simulink model "Control_Schematic_11"  (Simulink 8.3)
settings: Solver=ode4  StartTime=0.0  StopTime=50  FixedStep=Ts  RelTol=1e-3
values from neighbouring files (symbols this model uses):
  b = 156    [StartUp_1.m]    (also in StartUp_11_Validation.m; StartUp_3.m; StartUp_4.m; StartUp_7.m)
  r = 820    [StartUp_1.m]    (also in StartUp_11_Validation.m = 50; StartUp_3.m = 520; StartUp_4.m = 0.01; StartUp_7.m = 0.01)
  Ts = 1/1000    (= 0.001)    [StartUp_1.m]    (also in StartUp_11_Validation.m = 0.01; StartUp_3.m; StartUp_4.m; StartUp_7.m)
undefined symbols (not defined in the file or in its folder): Aob, Beta_Correction, Bob, Cob, Dob
undefined symbols (not defined in the file): ADAMS_cwd, ADAMS_exec, ADAMS_host, ADAMS_init, ADAMS_inputs, ADAMS_outputs, ADAMS_prefix, ADAMS_static, ADAMS_sysdir
libraries: cstblocks x2, simulink x1
settings Model: Creator=baqumau  LastModifiedBy=baqumau
settings DataIOCC: SignalLoggingSaveFormat=Dataset
settings DebuggingCC: UnderspecifiedInitializationDetection=Simplified  StateNameClashWarn=none
settings GRTTargetCC: CombineOutputUpdateFcns=on  GRTInterface=off

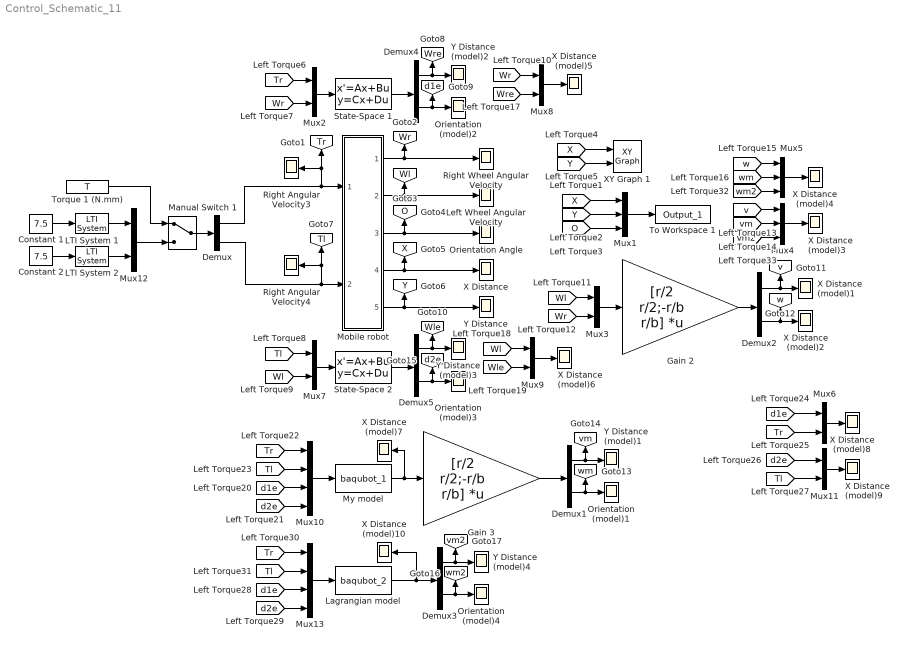
== system Control_Schematic_11 ==
  Constant 1 : Constant  Value=7.5
  Constant 2 : Constant  Value=7.5
  Demux{,1..5} (6 alike) : Demux  Outputs=2
  Gain 2 : Gain  Gain=[r/2 r/2;-r/b r/b]  Multiplication=Matrix(K*u)
  Gain 3 : Gain  Gain=[r/2 r/2;-r/b r/b]  Multiplication=Matrix(K*u)
  LTI System 1 : cstblocks/LTI System  sys=Fz  IC=[]
  LTI System 2 : cstblocks/LTI System  sys=Fz  IC=[]
  Lagrangian model : S-Function  FunctionName=baqubot_2  Parameters=par  EnableBusSupport=off
  Left Wheel Angular Velocity : Scope
      settings: YMin=-1  YMax=1  SaveName=ScopeData2
  Manual Switch 1 : ManualSwitch
  Mobile robot : Subsystem
  Mux1 : Mux  Inputs=3
  Mux10 : Mux
  Mux{2..3,6..9,11..12} (8 alike) : Mux  Inputs=2
  Mux13 : Mux
  Mux4 : Mux  Inputs=3
  Mux5 : Mux  Inputs=3
  My model : S-Function  FunctionName=baqubot_1  Parameters=par  EnableBusSupport=off
  Orientation (model){1..4} (4 alike) : Scope
      Orientation (model)1 settings: YMin=1.49226  YMax=1.64934  SaveName=ScopeData12
      Orientation (model)2 settings: YMin=-15  YMax=15  SaveName=ScopeData6
      Orientation (model)3 settings: YMin=-15  YMax=15  SaveName=ScopeData9
      Orientation (model)4 settings: YMin=1.49226  YMax=1.64934  SaveName=ScopeData23
  Orientation Angle : Scope
      settings: YMin=-4  YMax=4
  Right Angular Velocity3 : Scope
      settings: YMin=-1.5  YMax=5.5  SaveName=ScopeData7
  Right Angular Velocity4 : Scope
      settings: YMin=-25  YMax=25  SaveName=ScopeData8
  Right Wheel Angular Velocity : Scope
      settings: YMin=-1  YMax=1  SaveName=ScopeData3
  State-Space 1 : StateSpace  A=Aob  B=Bob  C=Cob  D=Dob  X0=0
  State-Space 2 : StateSpace  A=Aob  B=Bob  C=Cob  D=Dob  X0=0
  To Workspace 1 : ToWorkspace  VariableName=Output_1  SaveFormat=Structure With Time  SampleTime=-1
  Torque 1 (N.mm) : FromWorkspace  VariableName=T  SampleTime=Ts  Interpolate=off  OutputAfterFinalValue=Holding final value
  X Distance : Scope
      settings: YMin=0  YMax=5000  SaveName=ScopeData4
  X Distance (model){1..10} (10 alike) : Scope
      X Distance (model)1 settings: YMin=0  YMax=5000  SaveName=ScopeData10
      X Distance (model)10 settings: YMin=0  YMax=5000  SaveName=ScopeData22
      X Distance (model)2 settings: YMin=0  YMax=5000  SaveName=ScopeData11
      X Distance (model)3 settings: YMin=0  YMax=800  SaveName=ScopeData14
      X Distance (model)4 settings: YMin=0  YMax=5000  SaveName=ScopeData15
      X Distance (model)5 settings: YMin=0  YMax=5000  SaveName=ScopeData17
      X Distance (model)6 settings: YMin=0  YMax=5000  SaveName=ScopeData18
      X Distance (model)7 settings: YMin=0  YMax=5000  SaveName=ScopeData19
      X Distance (model)8 settings: TimeRange=35  YMin=-20  YMax=20  SaveName=ScopeData20
      X Distance (model)9 settings: YMin=-15  YMax=15  SaveName=ScopeData21
  XY Graph 1 : simulink/Sinks/XY Graph  xmin=0  xmax=5000  ymin=0  ymax=5000  st=-1
  Y Distance : Scope
      settings: YMin=0  YMax=5000
  Y Distance (model){1..4} (4 alike) : Scope
      Y Distance (model)1 settings: YMin=0  YMax=5000  SaveName=ScopeData13
      Y Distance (model)2 settings: YMin=0  YMax=5000  SaveName=ScopeData5
      Y Distance (model)3 settings: YMin=0  YMax=5000  SaveName=ScopeData16
      Y Distance (model)4 settings: YMin=0  YMax=5000  SaveName=ScopeData24
  tag scope: O=global, Tl=global, Tr=global, Wl=global, Wle=global, Wr=global, Wre=global, X=global, Y=global, d1e=global, d2e=global, v=global, vm2=global, vm=global, w=global, wm2=global, wm=global
  wires:
  Mobile robot/1(Wrw) -> Right Wheel Angular Velocity/1, [Wr]
  Mobile robot/2(Wlw) -> Left Wheel Angular Velocity/1, [Wl]
  Mobile robot/3(Alpha) -> Orientation Angle/1, [O]
  Mobile robot/4(X_Dist) -> X Distance/1, [X]
  Mobile robot/5(Y_Dist) -> Y Distance/1, [Y]
  [X] -> Mux1/1
  [Y] -> Mux1/2
  [O] -> Mux1/3
  Mux1/1 -> To Workspace 1/1
  Demux/1 -> Mobile robot/1(Trw), [Tr], Right Angular Velocity3/1
  Demux/2 -> Mobile robot/2(Tlw), [Tl], Right Angular Velocity4/1
  [X] -> XY Graph 1/1
  [Y] -> XY Graph 1/2
  [Wl] -> Mux3/1
  [Wr] -> Mux3/2
  Mux3/1 -> Gain 2/1
  Gain 2/1 -> Demux2/1
  Demux2/2 -> [w], X Distance (model)2/1
  Demux2/1 -> [v], X Distance (model)1/1
  Demux1/1 -> Y Distance (model)1/1, [vm]
  Demux1/2 -> Orientation (model)1/1, [wm]
  [vm] -> Mux4/2
  Mux4/1 -> X Distance (model)3/1
  [wm] -> Mux5/2
  Mux5/1 -> X Distance (model)4/1
  [Tr] -> Mux10/1
  Gain 3/1 -> Demux1/1
  Mux10/1 -> My model/1
  My model/1 -> X Distance (model)7/1, Gain 3/1
  Mux2/1 -> State-Space 1/1
  [Tr] -> Mux2/1
  [Wr] -> Mux2/2
  State-Space 1/1 -> Demux4/1
  Demux4/2 -> [d1e], Orientation (model)2/1
  Demux4/1 -> [Wre], Y Distance (model)2/1
  Mux7/1 -> State-Space 2/1
  [Tl] -> Mux7/1
  [Wl] -> Mux7/2
  State-Space 2/1 -> Demux5/1
  Demux5/2 -> Orientation (model)3/1, [d2e]
  Demux5/1 -> Y Distance (model)3/1, [Wle]
  [Wr] -> Mux8/1
  Mux8/1 -> X Distance (model)5/1
  [Wre] -> Mux8/2
  Mux9/1 -> X Distance (model)6/1
  [Wle] -> Mux9/2
  [Wl] -> Mux9/1
  [Tl] -> Mux10/2
  [d1e] -> Mux10/3
  [d2e] -> Mux10/4
  [d1e] -> Mux6/1
  [Tr] -> Mux6/2
  Mux6/1 -> X Distance (model)8/1
  [d2e] -> Mux11/1
  [Tl] -> Mux11/2
  Mux11/1 -> X Distance (model)9/1
  Manual Switch 1/1 -> Demux/1
  Torque 1 (N.mm)/1 -> Manual Switch 1/1
  Constant 1/1 -> LTI System 1/1
  Constant 2/1 -> LTI System 2/1
  LTI System 2/1 -> Mux12/2
  LTI System 1/1 -> Mux12/1
  Mux12/1 -> Manual Switch 1/2
  [Tr] -> Mux13/1
  Mux13/1 -> Lagrangian model/1
  [Tl] -> Mux13/2
  [d1e] -> Mux13/3
  [d2e] -> Mux13/4
  Demux3/1 -> [vm2], Y Distance (model)4/1
  Demux3/2 -> [wm2], Orientation (model)4/1
  Lagrangian model/1 -> X Distance (model)10/1, Demux3/1
  [wm2] -> Mux5/3
  [vm2] -> Mux4/3
  [w] -> Mux5/1
  [v] -> Mux4/1

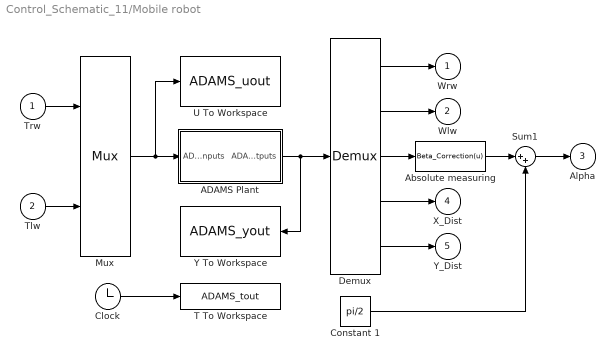
== system Control_Schematic_11/Mobile robot ==
  Trw : Inport
  Tlw : Inport  Port=2
  ADAMS Plant : Subsystem  LoadFcn=|  InitFcn=clear mex  mask(Adams Plant){exevie=ADAMS_sysdir, nam_in=ADAMS_inputs, namout=ADAMS_outputs, nampre=ADAMS_prefix, outfil=ADAMS_prefix, exesol=ADAMS_exec, stat=ADAMS_static, inicmd=[ADAMS_init], exetyp=C++, comtyp=PIPE(DDE), workdir=ADAMS_cwd, ada_host=ADAMS_host, modani=batch, modsim=discrete, dft=no, simulink_lead_cosim=yes, pin_interp_order=0, pout_extrap_order=0, pin_extrap_order=0, pout_interp_order=0, dt_out=Ts, o_rate=1, more=off}
      | %check based on dialog box setting for when setting by popup menu                                             
      | if exist('ADAMS_solver_type')                                                                                 
      |   if strcmp(ADAMS_solver_type,'C++')                                                                          
      |     set_param(gcb,'exetyp','C++');                                                                            
      |   else                                                                                                        
      |     set_param(gcb,'exetyp','Fortran');                                                                        
      |   end                                                                                                         
      | else                                                                                                          
      |   set_param(gcb,'exetyp','C++');                                                                              
      | end                                                                                                           
      | %set the mode if using acar_solver                                                                            
      | %REQUIRED HERE BECAUSE BELOW CAUSES MDLTERMINATE TO BE CALLED 2 TIMES IN MIDDLE OF SIMULATION WHEN SET IN MASK
      |                                                                                                               
      | %enable the direct feedthrough, sim mode, anim mode parameters by default                                     
      |                                                                                                               
      | if exist('set_some_params_states')                                                                            
      |                                                                                                               
      |   set_some_params_states({'dft','modsim','modani'},{'on','on','on'},'MaskEnables',gcb)                        
      |   %turn on direct feedthrough option                                                                          
      |   set_some_params_states({'dft'},{'on'},'MaskVisibilities',gcb)                                               
      |                                                                                                               
      |  end                                                                                                          
      |                                                                                                               
      |                                                                                                               
      | if exist('ADAMS_exec')                                                                                        
      |   if and(strcmp(get_param(gcb,'exesol'),'ADAMS_exec'),strcmp(ADAMS_exec,'acar_solver'))                       
      |     %set the sim mode to discrete -- only supported mode                                                      
      |     set_param(gcb,'modsim','discrete')                                                                        
      |      %turn off direct feedthrough option                                                                      
      |      set_some_params_states({'dft'},{'off'},'MaskVisibilities',gcb)                                           
      |     %set the animation mode to batch -- only supported mode                                                   
      |     set_param(gcb,'modani','batch')                                                                           
      |     %disable the direct feedthrough, sim mode, anim mode parameters                                           
      |     set_some_params_states({'modsim','modani'},{'off','off'},'MaskEnables',gcb)                               
      |   end                                                                                                         
      | end
      mask prompts: exevie "Adams install directory"; nam_in "Adams/View input names"; namout "Adams/View output names"; nampre "Adams model file prefix"; outfil "Output files prefix (opt.: if blank - no output)"; exesol "User executable (opt.: if blank - use standard)"; stat "Initial static simulation flag"; inicmd "Initialization commands"; exetyp "Adams/Solver type"; comtyp "Interprocess option"; workdir "Adams working directory"; ada_host "Adams host"; modani "Animation mode"; modsim "Simulation mode"; dft "Direct feedthrough"; simulink_lead_cosim "Discrete Computational Order - Simulink Leads Adams"; pin_interp_order "Plant input interpolation order"; pout_extrap_order "Plant output extrapolation order"; pin_extrap_order "Plant input extrapolation order"; pout_interp_order "Plant output interpolation order"; dt_out "Communication interval"; o_rate "Number of communications per output step"; more "More parameters"
      mask help: Simulate any Adams plant model either in Adams/Solver form (.adm file) or in Adams/View form (.cmd file)
      settings: OpenFcn=|
      | open_system(gcb,'mask')
      | if not(exist('set_some_params_states'))
      | 
      | warning('The script "set_some_params_states.m" cannot be found in the MATLAB PATH.  Cannot update the ADAMS Plant S-Function parameters.')
      | 
      | warning('Recommended action(optional):  run the Adams/Controls .m file first to help choose the correct settings in the Adams S-Function block.')
      | 
      | end
      mask Help:
      | <html>
      | This S-Function represents the non-linear Adams Plant with the inputs sent to the Adams model <br>
      |  and the outputs generated by the Adams model.  See the Adams/Controls documentation for more <br>
      | information.  This plant uses the following variables:<br>
      | <br>
      | <b>ADAMS_sysdir  :</b> Adams installation directory<br>
      | <b>ADAMS_inputs  :</b> Input variables View names vector<br>
      | <b>ADAMS_outputs :</b> Outputs variables View names vector<br>
      | <b>ADAMS_prefix  : </b>ADAMS model files prefix (.adm, .cmd); also doubles as output files prefix<br>
      | <b>ADAMS_exec :</b> Adams/Solver user library or keyword (e.g., acar_solver)<br>
      | <b>ADAMS_static :</b> yes|no - initial static before Co-simulation(discrete)/Function Evaluation(continuous)<br>
      | <b>ADAMS_init :</b>Initialization commands (i.e., Adams/View or Solver commands, depending on setting for Animation mode)<br>
      | <b>ADAMS_cwd : </b> Current working directory (for TCP/IP)<br>
      | <b>ADAMS_host : </b>Name of Adams server host (for TCP/IP)<br>
      | <b>ADAMS_mode :</b> Linear or non-linear (i.e., co-sim, function eval)<br>
      | <b>ADAMS_solver_type :</b>Fortran or C++ (used to set popup menu when first loaded) <br>
      | 
      | 
      | <br>
      | The following settings can be chosen:<br>
      | <br>
      | <b>Adams/Solver type:</b>  Fortran or C++ (will also set ADAMS_solver_type)<br>
      | <b>Interprocess option:</b> Pipe(DDE) or TCP/IP; TCP/IP can allow different machines run Adams and MATLAB<br>
      | <b>Animation mode:</b> batch (Solver, uses .adm) or interactive (View, uses .cmd)<br>
      | <b>Simulation mode:</b> discrete (Co-simulation) or continuous (Function Evaluation)<br>
      | <b>Discrete Computational Order - Simulink Lead Adams:</b> for discrete mode, chooses if Simulink leads the integration (yes) or lags (no);<br> if set to "no", can remove algebraic loop<br>
      | <b>Plant input interpolation order:</b> 0 = zero-order hold; 1 = linear (discrete mode only, where Simulink leads)<br>
      | <b>Plant output extrapolation order:</b> 0 = zero-order hold;1 = linear(discrete mode only, where Simulink leads)<br>
      | <b>Plant input extrapolation order:</b> 0 = zero-order hold; 1 = linear (discrete mode only, where Adams leads)<br>
      | <b>Plant output interpolation order:</b> 0 = zero-order hold;1 = linear(discrete mode only, where Adams leads)<br>
      | <b>Direct feedthrough:</b> yes|no - yes = Input directly effect output(continuous mode-only)<br>
      | <b>Communication interval:</b> Time step at which Co-simulation exchange information (e.g.,0.005); also controls <br>output for continuous mode (Function Evaluation)<br>
      | <b>Number of communications per output step: </b>Sets Adams output rate (.res, .req, .gra) integer value (default: 1)<br>
      | </html>
      mask Callback exesol:
      | if exist('set_some_params_states')
      | %enable the direct feedthrough, sim mode, anim mode parameters
      | set_some_params_states({'dft','modsim','modani'},{'on','on','on'},'MaskEnables',gcb)
      | %turn on direct feedthrough option
      | set_some_params_states({'dft'},{'on'},'MaskVisibilities',gcb)
      | end
      | 
      | if exist('ADAMS_exec')
      |   if and(strcmp(get_param(gcb,'exesol'),'ADAMS_exec'),strcmp(ADAMS_exec,'acar_solver'))
      |     %set the sim mode to discrete -- only supported mode
      |     %REMOVED:  BELOW CAUSES MDLTERMINATE TO BE CALLED 2 TIMES IN MIDDLE OF SIMULATION
      |     %Now in LoadFcn callback
      |     %set_param(gcb,'modsim','discrete')
      |      %turn off direct feedthrough option
      |     set_some_params_states({'dft'},{'off'},'MaskVisibilities',gcb)
      |     %set the animation mode to batch -- only supported mode
      |     %REMOVED:  BELOW CAUSES MDLTERMINATE TO BE CALLED 2 TIMES IN MIDDLE OF SIMULATION
      |     %Now in LoadFcn callback
      |     %set_param(gcb,'modani','batch')
      |     %disable the direct feedthrough, sim mode, anim mode parameters
      |     set_some_params_states({'modsim','modani'},{'off','off'},'MaskEnables',gcb)
      |   end
      | end
      mask TypeOptions exetyp: Fortran | C++
      mask Callback exetyp:
      | if strcmp(get_param(gcb,'exetyp'),'C++')
      |     ADAMS_solver_type='C++';
      | else
      |     ADAMS_solver_type='Fortran';
      | end
      mask TypeOptions comtyp: PIPE(DDE) | TCP/IP
      mask Callback comtyp:
      | if exist('set_some_params_states')
      | if strcmp(get_param(gcb,'comtyp'),'PIPE(DDE)')
      |     %turn off cwd, host options
      |     set_some_params_states({'ada_host','workdir'},{'off','off'},'MaskVisibilities',gcb)
      | else%if strcmp(get_param(gcb,'modsim'),'TCP/IP')
      |     %turn on cwd, host options
      |     set_some_params_states({'ada_host','workdir'},{'on','on'},'MaskVisibilities',gcb)
      | end
      | end
      mask TypeOptions modani: batch | interactive
      mask TypeOptions modsim: discrete | continuous
      mask Callback modsim:
      | if exist('set_some_params_states')
      | if strcmp(get_param(gcb,'modsim'),'discrete')
      |      %turn off direct feedthrough option
      |     set_some_params_states({'dft'},{'off'},'MaskVisibilities',gcb)
      |     %turn on discrete co-sim type if want to see more
      |     if strcmp(get_param(gcb,'more'),'on')
      |         set_some_params_states({'simulink_lead_cosim'},{'on'},'MaskVisibilities',gcb)
      |     end
      |     if strcmp(get_param(gcb,'simulink_lead_cosim'),'yes')
      |         %turn on interpolation/extrapolation options
      |         set_some_params_states({'pin_interp_order','pout_extrap_order',},{'on','on'},'MaskVisibilities',gcb)
      |     else
      |         set_some_params_states({'pin_extrap_order','pout_interp_order'},{'on','on'},'MaskVisibilities',gcb)
      |     end
      | else%if strcmp(get_param(gcb,'modsim'),'continuous')
      |      %turn off direct feedthrough option
      |     set_some_params_states({'dft'},{'on'},'MaskVisibilities',gcb)
      |     %turn off interpolation/extrapolation options
      |     set_some_params_states({'pin_interp_order','pout_extrap_order','pin_extrap_order','pout_interp_order','simulink_lead_cosim'},{'off','off','off','off','off'},'MaskVisibilities',gcb)
      | end
      | end
      mask TypeOptions dft: no | yes
      mask TypeOptions simulink_lead_cosim: yes | no
      mask Callback simulink_lead_cosim:
      | if exist('set_some_params_states')
      | if (strcmp(get_param(gcb,'simulink_lead_cosim'),'yes') && strcmp(get_param(gcb,'modsim'),'discrete'))
      |      %turn off unused interpolate/extrapolate options
      |     set_some_params_states({'pin_extrap_order','pout_interp_order'},{'off','off'},'MaskVisibilities',gcb)
      |     %turn on used interpolate/extrapolate options
      |     set_some_params_states({'pin_interp_order','pout_extrap_order'},{'on','on'},'MaskVisibilities',gcb)
      | elseif (strcmp(get_param(gcb,'simulink_lead_cosim'),'no') && strcmp(get_param(gcb,'modsim'),'discrete'))
      |     %turn on used interpolate/extrapolate options
      |     set_some_params_states({'pin_extrap_order','pout_interp_order'},{'on','on'},'MaskVisibilities',gcb)
      |      %turn off unused interpolate/extrapolate options
      |     set_some_params_states({'pin_interp_order','pout_extrap_order'},{'off','off'},'MaskVisibilities',gcb)
      | end
      | end
      mask TypeOptions pin_interp_order: 0 | 1
      mask TypeOptions pout_extrap_order: 0 | 1
      mask TypeOptions pin_extrap_order: 0 | 1
      mask TypeOptions pout_interp_order: 0 | 1
      mask Callback more:
      | if exist('set_some_params_states')
      | if (strcmp(get_param(gcb,'more'),'on'))
      |      %turn on infrequently used options
      |     set_some_params_states({'exevie','nam_in','namout','exesol','stat','inicmd'},{'on','on','on','on','on','on'},'MaskVisibilities',gcb)
      |     if strcmp(get_param(gcb,'modsim'),'discrete')
      |         set_some_params_states({'simulink_lead_cosim'},{'on'},'MaskVisibilities',gcb)
      |     end
      | elseif (strcmp(get_param(gcb,'more'),'off'))
      |     %turn off infrequently used options
      |     set_some_params_states({'exevie','nam_in','namout','exesol','stat','inicmd'},{'off','off','off','off','off','off'},'MaskVisibilities',gcb)
      |     if strcmp(get_param(gcb,'modsim'),'discrete')
      |         set_some_params_states({'simulink_lead_cosim'},{'off'},'MaskVisibilities',gcb)
      |     end
      | end
      | end
      mask Display: disp( 'MSC Software' )
  Absolute measuring : MATLABFcn  MATLABFcn=Beta_Correction(u)
  Clock : Clock
  Constant 1 : Constant  Value=pi/2
  Demux : Demux  Outputs=5
  Mux : Mux  Inputs=2
  Sum1 : Sum  Inputs=|++
  T To Workspace : ToWorkspace  VariableName=ADAMS_tout
      settings: MaxDataPoints=100000
  U To Workspace : ToWorkspace  VariableName=ADAMS_uout
      settings: MaxDataPoints=100000
  Y To Workspace : ToWorkspace  VariableName=ADAMS_yout
      settings: MaxDataPoints=100000
  Wrw : Outport
  Wlw : Outport  Port=2
  Alpha : Outport  Port=3
  X_Dist : Outport  Port=4
  Y_Dist : Outport  Port=5
  wires:
  Tlw/1 -> Mux/2
  Trw/1 -> Mux/1
  Demux/5 -> Y_Dist/1
  Demux/4 -> X_Dist/1
  Demux/2 -> Wlw/1
  Demux/1 -> Wrw/1
  ADAMS Plant/1(ADAMS outputs) -> Y To Workspace/1, Demux/1
  Mux/1 -> U To Workspace/1, ADAMS Plant/1(ADAMS inputs)
  Clock/1 -> T To Workspace/1
  Demux/3 -> Absolute measuring/1
  Absolute measuring/1 -> Sum1/1
  Constant 1/1 -> Sum1/2
  Sum1/1 -> Alpha/1

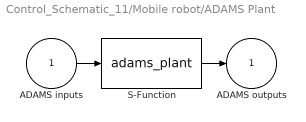
== system Control_Schematic_11/Mobile robot/ADAMS Plant ==
  ADAMS inputs : Inport
  S-Function : S-Function  StopFcn=clear mex  FunctionName=adams_plant  Parameters=exevie,exesol,stat,outfil,nampre,o_rate,nam_in,namout,dft,modsim,modani,dt_out,inicmd,exetyp,comtyp,ada_host, workdir,pin_interp_order,pout_extrap_order,pin_extrap_order,pout_interp_order,simulink_lead_cosim  EnableBusSupport=off
  ADAMS outputs : Outport  InitialOutput=0
  wires:
  S-Function/1 -> ADAMS outputs/1
  ADAMS inputs/1 -> S-Function/1
